simulink model "Poject_PilotInLoop_Beech_99_Nonlinear_Simulation_Altitude_hold"  (R2018b)
settings: Solver=FixedStepAuto  StartTime=0.0  StopTime=2144  FixedStep=0.01  RelTol=1e-3
InitFcn:
  | Initial_Data_Altitude_Hold
StopFcn:
  | Plots_Altitude_Hold
values from neighbouring files (symbols this model uses):
  b = 46    [Initial_Data_Altitude_Hold.m]    (also in TrimFunc.m)
  c = 6.5    [Initial_Data_Altitude_Hold.m]    (also in TrimFunc.m)
  CD0 = 0.0270    (= 0.027)    [Initial_Data_Altitude_Hold.m]    (also in TrimFunc.m)
  CDalpha = 0.131    [Initial_Data_Altitude_Hold.m]    (also in TrimFunc.m)
  CDalphadot = 0    [Initial_Data_Altitude_Hold.m]
  CDdelE = 0    [Initial_Data_Altitude_Hold.m]    (also in TrimFunc.m)
  CDiH = 0    [Initial_Data_Altitude_Hold.m]    (also in TrimFunc.m)
  CDq = 0    [Initial_Data_Altitude_Hold.m]
  CDu = 0    [Initial_Data_Altitude_Hold.m]
  CL0 = 0.201    [Initial_Data_Altitude_Hold.m]    (also in TrimFunc.m)
  CLalpha = 5.48    [Initial_Data_Altitude_Hold.m]    (also in TrimFunc.m)
  CLalphadot = 2.5    [Initial_Data_Altitude_Hold.m]
  Clbeta = -0.13    [Initial_Data_Altitude_Hold.m]    (also in TrimFunc.m)
  Clbetadot = 0    [Initial_Data_Altitude_Hold.m]
  CldelA = 0.156    [Initial_Data_Altitude_Hold.m]
  CLdelE = 0.60    (= 0.6)    [Initial_Data_Altitude_Hold.m]    (also in TrimFunc.m)
  CldelR = 0.0106    [Initial_Data_Altitude_Hold.m]    (also in TrimFunc.m)
  CLiH = 1.35    [Initial_Data_Altitude_Hold.m]    (also in TrimFunc.m)
  Clp = -0.50    (= -0.5)    [Initial_Data_Altitude_Hold.m]
  CLq = 8.1    [Initial_Data_Altitude_Hold.m]
  Clr = 0.14    [Initial_Data_Altitude_Hold.m]
  ClT = 0    [Initial_Data_Altitude_Hold.m]
  CLu = 0.020    (= 0.02)    [Initial_Data_Altitude_Hold.m]
  Cm0 = 0.05    [Initial_Data_Altitude_Hold.m]    (also in TrimFunc.m)
  Cmalpha = -1.89    [Initial_Data_Altitude_Hold.m]    (also in TrimFunc.m)
  Cmalphadot = -9.1    [Initial_Data_Altitude_Hold.m]
  CmdelE = -2.0    (= -2)    [Initial_Data_Altitude_Hold.m]    (also in TrimFunc.m)
  cmiH = -4.1    [Initial_Data_Altitude_Hold.m]
  Cmq = -34.0    (= -34)    [Initial_Data_Altitude_Hold.m]
  CmT1 = 0    [Initial_Data_Altitude_Hold.m]
  CmTalpha = 0    [Initial_Data_Altitude_Hold.m]
  CmTu = 0    [Initial_Data_Altitude_Hold.m]
  Cmu = 0    [Initial_Data_Altitude_Hold.m]
  Cnbeta = 0.080    (= 0.08)    [Initial_Data_Altitude_Hold.m]    (also in TrimFunc.m)
  Cnbetadot = 0    [Initial_Data_Altitude_Hold.m]
  CndelA = -0.0012    [Initial_Data_Altitude_Hold.m]    (also in TrimFunc.m)
  CndelR = -0.0758    [Initial_Data_Altitude_Hold.m]    (also in TrimFunc.m)
  Cnp = 0.019    [Initial_Data_Altitude_Hold.m]
  Cnr = -0.197    [Initial_Data_Altitude_Hold.m]
  CnTbeta = 0    [Initial_Data_Altitude_Hold.m]
  CTxu = -0.0596    [Initial_Data_Altitude_Hold.m]
  CTy = 0    [Initial_Data_Altitude_Hold.m]
  CTz = 0    [Initial_Data_Altitude_Hold.m]
  Cybeta = -0.59    [Initial_Data_Altitude_Hold.m]
  Cybetadot = 0    [Initial_Data_Altitude_Hold.m]
  CydelA = 0    [Initial_Data_Altitude_Hold.m]
  CydelR = 0.144    [Initial_Data_Altitude_Hold.m]
  Cyp = -0.19    [Initial_Data_Altitude_Hold.m]
  Cyr = 0.39    [Initial_Data_Altitude_Hold.m]
  delE = 0.0077075    [Initial_Data_Altitude_Hold.m]
  g = 32.17    [Initial_Data_Altitude_Hold.m]
  iH = 0    [Initial_Data_Altitude_Hold.m]    (also in TrimFunc.m)
  Ixx = 15189    [Initial_Data_Altitude_Hold.m]
  Ixz = 4371    [Initial_Data_Altitude_Hold.m]
  Iyy = 20250    [Initial_Data_Altitude_Hold.m]
  Izz = 34141    [Initial_Data_Altitude_Hold.m]
  Kp = 1    [Initial_Data_Altitude_Hold.m]
  mass = 341.9    [Initial_Data_Altitude_Hold.m]
  Ro = 0.0013    [Initial_Data_Altitude_Hold.m]
  S = 280    [Initial_Data_Altitude_Hold.m]    (also in TrimFunc.m)
  T1 = 1055.4173    [Initial_Data_Altitude_Hold.m]
  taw = 0.1    [Initial_Data_Altitude_Hold.m]
  TI = 0.2    [Initial_Data_Altitude_Hold.m]
  TL = 0.4    [Initial_Data_Altitude_Hold.m]
  TN = 0.1    [Initial_Data_Altitude_Hold.m]
libraries: simulink x1
(part 1 of 2)
settings Model: Creator=Mehdi RJ  LastModifiedBy=User
settings DataIOCC: LimitDataPoints=on  SaveFormat=Array  SignalLoggingSaveFormat=ModelDataLogs
settings OptimizationCC: BlockReduction=off  BooleanDataType=off  LifeSpan=inf
settings DebuggingCC: SaveWithParameterizedLinksMsg=none  UnderspecifiedInitializationDetection=Classic  MergeDetectMultiDrivingBlocksExec=none  SignalResolutionControl=TryResolveAllWithWarning  MultiTaskDSMMsg=warning  MultiTaskCondExecSysMsg=none  SFUnexpectedBacktrackingDiag=warning  SFNoUnconditionalDefaultTransitionDiag=warning  SFExecutionAtInitializationDiag=none
settings HardwareCC: ProdBitPerPointer=32  ProdBitPerSizeT=32  ProdBitPerPtrDiffT=32  ProdLargestAtomicFloat=None  ProdIntDivRoundTo=Undefined  ProdEndianess=Unspecified  ProdWordSize=32  ProdHWDeviceType=32-bit Generic  TargetUnknown=on
settings ModelReferenceCC: PropagateSignalLabelsOutOfModel=off
settings SFSimCC: SimUseLocalCustomCode=off
settings RTWCC: RTWUseLocalCustomCode=off
settings CodeAppCC: StateflowObjectComments=on
settings GRTTargetCC: TargetLangStandard=C89/C90 (ANSI)  GeneratePreprocessorConditionals=Disable all
settings ConfigComp: CovMetricSettings=dw  CovHtmlReporting=on  CovSaveCumulativeToWorkspaceVar=on  CovSaveSingleToWorkspaceVar=on  CovExternalEMLEnable=off

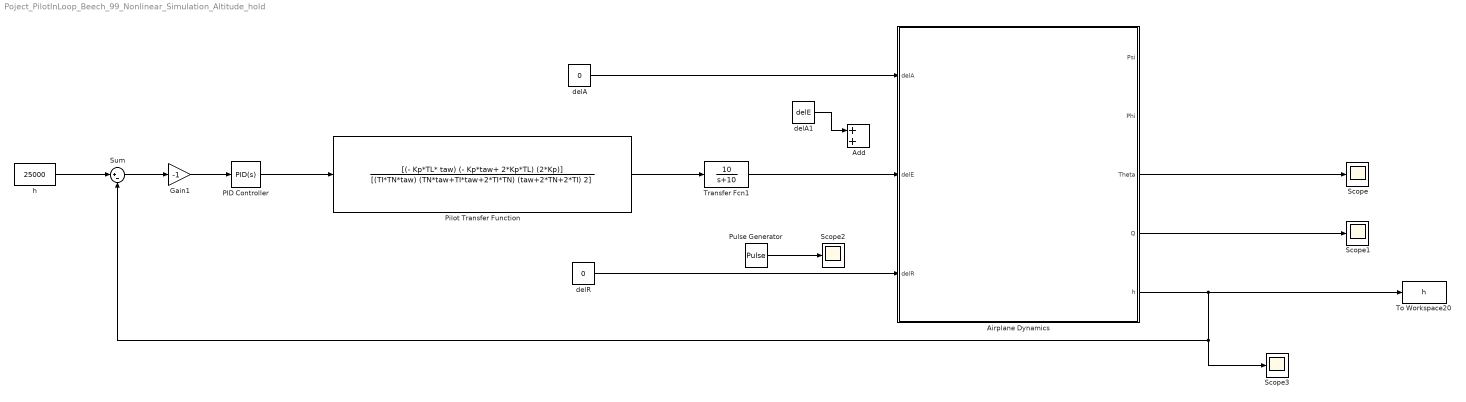
== system Poject_PilotInLoop_Beech_99_Nonlinear_Simulation_Altitude_hold ==
  Add : Sum
  Airplane Dynamics : Subsystem
  Gain1 : Gain  Gain=-1
  PID Controller : simulink/Continuous/PID Controller  Controller=PID  Form=Parallel  TimeDomain=Continuous-time  SampleTime=-1  IntegratorMethod=Forward Euler  FilterMethod=Forward Euler  ControllerParametersSource=internal  P=9.72091586765638e-06  I=5.86209894111036e-08  D=9.64251086658951e-05  UseFilter=on  N=15.2377063472214  TunerSelectOption=Transfer Function Based (PID Tuner App)  InitialConditionSource=internal  InitialConditionForIntegrator=0  InitialConditionForFilter=0  DifferentiatorICPrevScaledInput=0  ExternalReset=none  TrackingMode=off  Kt=1  LimitOutput=off  UpperSaturationLimit=inf  LowerSaturationLimit=-inf  LinearizeAsGain=on  AntiWindupMode=none  Kb=1  POutMin=[]  POutMax=[]  IOutMin=[]  IOutMax=[]  DOutMin=[]  DOutMax=[]  NOutMin=[]  NOutMax=[]  SumOutMin=[]  SumOutMax=[]  SaturationOutMin=[]  SaturationOutMax=[]  PParamMin=[]  PParamMax=[]  IParamMin=[]  IParamMax=[]  DParamMin=[]  DParamMax=[]  NParamMin=[]  NParamMax=[]  KbParamMin=[]  KbParamMax=[]  KtParamMin=[]  KtParamMax=[]  KbOutMin=[]  KbOutMax=[]  KtOutMin=[]  KtOutMax=[]  IntegratorOutMin=[]  IntegratorOutMax=[]  FilterOutMin=[]  FilterOutMax=[]  SumI1OutMin=[]  SumI1OutMax=[]  SumI2OutMin=[]  SumI2OutMax=[]  SumI3OutMin=[]  SumI3OutMax=[]  SumI4OutMin=[]  SumI4OutMax=[]  SumDOutMin=[]  SumDOutMax=[]  DifferentiatorOutMin=[]  DifferentiatorOutMax=[]  FilterDiffOutCoefMin=[]  FilterDiffOutCoefMax=[]  ReciprocalOutMin=[]  ReciprocalOutMax=[]  SumDenOutMin=[]  SumDenOutMax=[]  SumNumOutMin=[]  SumNumOutMax=[]  DivideOutMin=[]  DivideOutMax=[]  IntegratorContinuousStateAttributes=''  IntegratorStateMustResolveToSignalObject=off  IntegratorRTWStateStorageClass=Auto  FilterContinuousStateAttributes=''  FilterStateMustResolveToSignalObject=off  FilterRTWStateStorageClass=Auto  ParallelPVariant=InternalParameters  IdealPVariant=Disabled  IVariant=InternalParameters  DVariant=InternalParameters  IntegratorVariant=Continuous  SatVariant=Disabled  AWVariant=Passthrough  PCopyVariant=Disabled  TRVariant=Disabled  FdbkBlocksVariant=Forward  IdealPFdbkVariant=Disabled  SatFdbkVariant=Disabled  DerivativeFilterVariant=ContFilter  NVariant=InternalParameters  NCopyVariant=Disabled  FilterICVariant=InternalICsFilter  IntegratorICVariant=InternalICs  ExternalResetVariant=Disabled  TRSumVariant=Passthrough  SumFdbkVariant=Disabled  SumVariant=Sum_PID
  Pilot Transfer Function : TransferFcn  Numerator=[(- Kp*TL* taw) (- Kp*taw+ 2*Kp*TL) (2*Kp)]  Denominator=[(TI*TN*taw) (TN*taw+TI*taw+2*TI*TN) (taw+2*TN+2*TI) 2]
  Pulse Generator : DiscretePulseGenerator  PulseType=Time based  Amplitude=0.0175*5  Period=2000  PhaseDelay=800
  Scope{,1..3} (4 alike) : Scope
  Sum : Sum  Inputs=|+-
  To Workspace20 : ToWorkspace  VariableName=h  SampleTime=-1
  Transfer Fcn1 : TransferFcn  Numerator=[10]  Denominator=[1 10]
  delA : Constant  Value=0
  delA1 : Constant  Value=delE
  delR : Constant  Value=0
  h : Constant  Value=25000
  wires:
  delR/1 -> Airplane Dynamics/3(delR)
  delA/1 -> Airplane Dynamics/1(delA)
  Airplane Dynamics/3(Theta) -> Scope/1
  h/1 -> Sum/1
  Airplane Dynamics/4(Q) -> Scope1/1
  Pulse Generator/1 -> Scope2/1
  Sum/1 -> Gain1/1
  Gain1/1 -> PID Controller/1
  Airplane Dynamics/5(h) -> Sum/2, Scope3/1, To Workspace20/1
  Pilot Transfer Function/1 -> Transfer Fcn1/1
  PID Controller/1 -> Pilot Transfer Function/1
  delA1/1 -> Add/1
  Transfer Fcn1/1 -> Airplane Dynamics/2(delE)

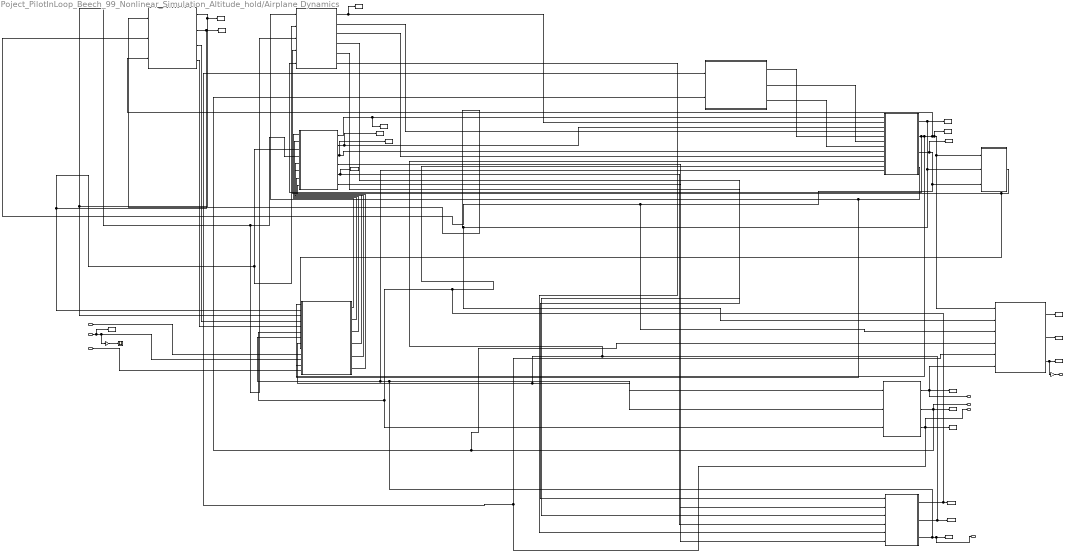
== system Poject_PilotInLoop_Beech_99_Nonlinear_Simulation_Altitude_hold/Airplane Dynamics ==
  delA : Inport
  delE : Inport  Port=2
  delR : Inport  Port=3
  AnglesBlock : Subsystem
  Angular Velocities (P,Q,R) : Subsystem
  Body Aerodynamic Forces and Moments (FAxB,FAyB,FAzB,LAB,MAB,NAB) : Subsystem
  Dynamic Pressure : Subsystem
  Euler's Angles (Phi,Theta,Psi) : Subsystem
  GBlock : Subsystem
  Gain : Gain  Gain=-1
  Gain1 : Gain  Gain=180/pi
  Linear Velocities (U,V,W) : Subsystem
  Navigation : Subsystem
  Scope : Scope
  Stability Aerodunamic Forces and Moments (FAxS,FAyS,FAzS,LAS,MAS,NAS) : Subsystem
  Thrust Forces and Moments (FTx,FTy,FTz,LT,MT,NT) : Subsystem
  To Workspace : ToWorkspace  VariableName=XInertia  SampleTime=-1
  To Workspace1 : ToWorkspace  VariableName=YInertia  SampleTime=-1
  To Workspace10 : ToWorkspace  VariableName=Q  SaveFormat=Timeseries  SampleTime=-1
  To Workspace11 : ToWorkspace  VariableName=R  SaveFormat=Timeseries  SampleTime=-1
  To Workspace12 : ToWorkspace  VariableName=P  SaveFormat=Timeseries  SampleTime=-1
  To Workspace13 : ToWorkspace  VariableName=W  SaveFormat=Timeseries  SampleTime=-1
  To Workspace14 : ToWorkspace  VariableName=FAzB  SaveFormat=Timeseries  SampleTime=-1
  To Workspace15 : ToWorkspace  VariableName=FTx  SaveFormat=Timeseries  SampleTime=-1
  To Workspace16 : ToWorkspace  VariableName=FAxB  SaveFormat=Timeseries  SampleTime=-1
  To Workspace17 : ToWorkspace  VariableName=FAyB  SaveFormat=Timeseries  SampleTime=-1
  To Workspace18 : ToWorkspace  VariableName=V  SaveFormat=Timeseries  SampleTime=-1
  To Workspace19 : ToWorkspace  VariableName=delE  SaveFormat=Timeseries  SampleTime=-1
  To Workspace2 : ToWorkspace  VariableName=ZInertia  SaveFormat=Timeseries  SampleTime=-1
  To Workspace3 : ToWorkspace  VariableName=alpha  SaveFormat=Timeseries  SampleTime=-1
  To Workspace4 : ToWorkspace  VariableName=beta  SaveFormat=Timeseries  SampleTime=-1
  To Workspace5 : ToWorkspace  VariableName=U  SaveFormat=Timeseries  SampleTime=-1
  To Workspace6 : ToWorkspace  VariableName=Psi  SaveFormat=Timeseries  SampleTime=-1
  To Workspace7 : ToWorkspace  VariableName=Phi  SaveFormat=Timeseries  SampleTime=-1
  To Workspace8 : ToWorkspace  VariableName=Theta  SaveFormat=Timeseries  SampleTime=-1
  To Workspace9 : ToWorkspace  VariableName=MAB  SaveFormat=Timeseries  SampleTime=-1
  Psi : Outport
  Phi : Outport  Port=2
  Theta : Outport  Port=3
  Q : Outport  Port=4
  h : Outport  Port=5
  wires:
  AnglesBlock/2(alpha) -> To Workspace3/1, Thrust Forces and Moments (FTx,FTy,FTz,LT,MT,NT)/2(alpha), Body Aerodynamic Forces and Moments (FAxB,FAyB,FAzB,LAB,MAB,NAB)/3(alpha), Stability Aerodunamic Forces and Moments (FAxS,FAyS,FAzS,LAS,MAS,NAS)/2(alpha)
  Stability Aerodunamic Forces and Moments (FAxS,FAyS,FAzS,LAS,MAS,NAS)/1(FAxS) -> Body Aerodynamic Forces and Moments (FAxB,FAyB,FAzB,LAB,MAB,NAB)/1(FAxS)
  Thrust Forces and Moments (FTx,FTy,FTz,LT,MT,NT)/2(FTy) -> Linear Velocities (U,V,W)/4(FTy)
  Thrust Forces and Moments (FTx,FTy,FTz,LT,MT,NT)/5(MT) -> Angular Velocities (P,Q,R)/3(MT)
  Angular Velocities (P,Q,R)/1(P) -> To Workspace12/1, Linear Velocities (U,V,W)/11(P), Stability Aerodunamic Forces and Moments (FAxS,FAyS,FAzS,LAS,MAS,NAS)/6(P), Euler's Angles (Phi,Theta,Psi)/3(P)
  AnglesBlock/3(betadot) -> Stability Aerodunamic Forces and Moments (FAxS,FAyS,FAzS,LAS,MAS,NAS)/4("betadot ")
  Euler's Angles (Phi,Theta,Psi)/1(Psi) -> To Workspace6/1, Navigation/6(Psi), Psi/1
  delR/1 -> Stability Aerodunamic Forces and Moments (FAxS,FAyS,FAzS,LAS,MAS,NAS)/13(delR)
  Body Aerodynamic Forces and Moments (FAxB,FAyB,FAzB,LAB,MAB,NAB)/4(LAB) -> Angular Velocities (P,Q,R)/2(LAB)
  Body Aerodynamic Forces and Moments (FAxB,FAyB,FAzB,LAB,MAB,NAB)/5(MAB) -> To Workspace9/1, Angular Velocities (P,Q,R)/4(MAB)
  Linear Velocities (U,V,W)/3(W) -> To Workspace13/1, Dynamic Pressure/3(W), AnglesBlock/2(W), Navigation/3(W)
  Angular Velocities (P,Q,R)/3(Q) -> Euler's Angles (Phi,Theta,Psi)/2(Q), Linear Velocities (U,V,W)/12(Q), Stability Aerodunamic Forces and Moments (FAxS,FAyS,FAzS,LAS,MAS,NAS)/7(Q), Q/1, To Workspace10/1
  Linear Velocities (U,V,W)/1(V) -> To Workspace18/1, Dynamic Pressure/2(V), AnglesBlock/1(V), Navigation/2(V)
  Euler's Angles (Phi,Theta,Psi)/3(Theta) -> To Workspace8/1, GBlock/1(Theta), Navigation/5(Theta), Theta/1
  AnglesBlock/1("beta ") -> To Workspace4/1, Body Aerodynamic Forces and Moments (FAxB,FAyB,FAzB,LAB,MAB,NAB)/4(beta), Thrust Forces and Moments (FTx,FTy,FTz,LT,MT,NT)/3(beta), Stability Aerodunamic Forces and Moments (FAxS,FAyS,FAzS,LAS,MAS,NAS)/3(beta)
  Linear Velocities (U,V,W)/4(delU) -> Stability Aerodunamic Forces and Moments (FAxS,FAyS,FAzS,LAS,MAS,NAS)/1(delU), Thrust Forces and Moments (FTx,FTy,FTz,LT,MT,NT)/1(delU)
  Thrust Forces and Moments (FTx,FTy,FTz,LT,MT,NT)/3(FTz) -> Linear Velocities (U,V,W)/9(FTz)
  Navigation/2(YInertia) -> To Workspace1/1
  Stability Aerodunamic Forces and Moments (FAxS,FAyS,FAzS,LAS,MAS,NAS)/4(LAS) -> Body Aerodynamic Forces and Moments (FAxB,FAyB,FAzB,LAB,MAB,NAB)/6(LAS)
  Euler's Angles (Phi,Theta,Psi)/2(Phi) -> To Workspace7/1, Navigation/4(Phi), GBlock/2("Phi "), Phi/1
  Body Aerodynamic Forces and Moments (FAxB,FAyB,FAzB,LAB,MAB,NAB)/3(FAzB) -> To Workspace14/1, Linear Velocities (U,V,W)/8(FAzB)
  Stability Aerodunamic Forces and Moments (FAxS,FAyS,FAzS,LAS,MAS,NAS)/2(FAyS) -> Body Aerodynamic Forces and Moments (FAxB,FAyB,FAzB,LAB,MAB,NAB)/2(FAyS)
  GBlock/2(gy) -> Linear Velocities (U,V,W)/6(gy)
  AnglesBlock/4(alphadot) -> Stability Aerodunamic Forces and Moments (FAxS,FAyS,FAzS,LAS,MAS,NAS)/5(alphadot)
  Navigation/1(XInertia) -> To Workspace/1
  Thrust Forces and Moments (FTx,FTy,FTz,LT,MT,NT)/1(FTx) -> To Workspace15/1, Linear Velocities (U,V,W)/2(FTx)
  Stability Aerodunamic Forces and Moments (FAxS,FAyS,FAzS,LAS,MAS,NAS)/5(MAS) -> Body Aerodynamic Forces and Moments (FAxB,FAyB,FAzB,LAB,MAB,NAB)/7(MAS)
  Thrust Forces and Moments (FTx,FTy,FTz,LT,MT,NT)/6(NT) -> Angular Velocities (P,Q,R)/5(NT)
  Stability Aerodunamic Forces and Moments (FAxS,FAyS,FAzS,LAS,MAS,NAS)/6(NAS) -> Body Aerodynamic Forces and Moments (FAxB,FAyB,FAzB,LAB,MAB,NAB)/8(NAS)
  Navigation/3(ZInertia) -> Gain/1, To Workspace2/1
  Linear Velocities (U,V,W)/2(U) -> Thrust Forces and Moments (FTx,FTy,FTz,LT,MT,NT)/5(U), Stability Aerodunamic Forces and Moments (FAxS,FAyS,FAzS,LAS,MAS,NAS)/12(U), AnglesBlock/3(U), To Workspace5/1, Navigation/1(U), Dynamic Pressure/1(U)
  Stability Aerodunamic Forces and Moments (FAxS,FAyS,FAzS,LAS,MAS,NAS)/3(FAzS) -> Body Aerodynamic Forces and Moments (FAxB,FAyB,FAzB,LAB,MAB,NAB)/5(FAzS)
  Dynamic Pressure/1(q1) -> Stability Aerodunamic Forces and Moments (FAxS,FAyS,FAzS,LAS,MAS,NAS)/9(q1), Thrust Forces and Moments (FTx,FTy,FTz,LT,MT,NT)/4(q1)
  Body Aerodynamic Forces and Moments (FAxB,FAyB,FAzB,LAB,MAB,NAB)/6(NAB) -> Angular Velocities (P,Q,R)/6(NAB)
  GBlock/1(gx) -> Linear Velocities (U,V,W)/5(gx)
  GBlock/3(gz) -> Linear Velocities (U,V,W)/7(gz)
  Body Aerodynamic Forces and Moments (FAxB,FAyB,FAzB,LAB,MAB,NAB)/1(FAxB) -> To Workspace16/1, Linear Velocities (U,V,W)/1(FAxB)
  Angular Velocities (P,Q,R)/2(R) -> To Workspace11/1, Stability Aerodunamic Forces and Moments (FAxS,FAyS,FAzS,LAS,MAS,NAS)/8(R), Euler's Angles (Phi,Theta,Psi)/1(R), Linear Velocities (U,V,W)/10(R)
  Thrust Forces and Moments (FTx,FTy,FTz,LT,MT,NT)/4(LT) -> Angular Velocities (P,Q,R)/1(LT)
  Body Aerodynamic Forces and Moments (FAxB,FAyB,FAzB,LAB,MAB,NAB)/2(FAyB) -> To Workspace17/1, Linear Velocities (U,V,W)/3(FAyB)
  delA/1 -> Stability Aerodunamic Forces and Moments (FAxS,FAyS,FAzS,LAS,MAS,NAS)/10(delA)
  Gain/1 -> h/1
  delE/1 -> To Workspace19/1, Gain1/1, Stability Aerodunamic Forces and Moments (FAxS,FAyS,FAzS,LAS,MAS,NAS)/11(delE)
  Gain1/1 -> Scope/1

== system Poject_PilotInLoop_Beech_99_Nonlinear_Simulation_Altitude_hold/Airplane Dynamics/AnglesBlock ==
  V : Inport
  W : Inport  Port=2
  U : Inport  Port=3
  Atan2 : Trigonometry  Operator=atan2
  Derivative : Derivative
  Derivative1 : Derivative
  Divide : Product  Inputs=*/
  Scope : Scope
  Sin : Trigonometry  Operator=asin
  "beta " : Outport
  alpha : Outport  Port=2
  betadot : Outport  Port=3
  alphadot : Outport  Port=4
  wires:
  U/1 -> Atan2/2, Divide/2
  W/1 -> Atan2/1
  V/1 -> Divide/1
  Atan2/1 -> Derivative1/1, Scope/1, alpha/1
  Sin/1 -> Derivative/1, "beta "/1
  Divide/1 -> Sin/1
  Derivative/1 -> betadot/1
  Derivative1/1 -> alphadot/1

== system Poject_PilotInLoop_Beech_99_Nonlinear_Simulation_Altitude_hold/Airplane Dynamics/Angular Velocities (P,Q,R) ==
  LT : Inport
  LAB : Inport  Port=2
  MT : Inport  Port=3
  MAB : Inport  Port=4
  NT : Inport  Port=5
  NAB : Inport  Port=6
  PBlock : Subsystem
  QBlock : Subsystem
  RBlock : Subsystem
  Scope : Scope
  P : Outport
  R : Outport  Port=2
  Q : Outport  Port=3
  wires:
  PBlock/2(Pdot) -> RBlock/3(Pdot)
  PBlock/1(P) -> RBlock/5(P), QBlock/3(P), P/1
  RBlock/2("Rdot ") -> PBlock/3(Rdot)
  LT/1 -> PBlock/2(LT)
  MAB/1 -> QBlock/1(MAB)
  LAB/1 -> PBlock/1(LAB)
  RBlock/1(R) -> R/1, PBlock/4(R), QBlock/4(R)
  NAB/1 -> RBlock/1(NAB)
  NT/1 -> RBlock/2(NT)
  MT/1 -> QBlock/2(MT)
  QBlock/1(Q) -> PBlock/5(Q), RBlock/4(Q), Scope/1, Q/1

== system Poject_PilotInLoop_Beech_99_Nonlinear_Simulation_Altitude_hold/Airplane Dynamics/Body Aerodynamic Forces and Moments (FAxB,FAyB,FAzB,LAB,MAB,NAB) ==
  FAxS : Inport
  FAyS : Inport  Port=2
  alpha : Inport  Port=3
  beta : Inport  Port=4
  FAzS : Inport  Port=5
  LAS : Inport  Port=6
  MAS : Inport  Port=7
  NAS : Inport  Port=8
  FAxBBlock : Subsystem
  FAyBBlock : Subsystem
  FAzBBlock : Subsystem
  LABBlock : Subsystem
  MABBlock : Subsystem
  NABBlock : Subsystem
  FAxB : Outport
  FAyB : Outport  Port=2
  FAzB : Outport  Port=3
  LAB : Outport  Port=4
  MAB : Outport  Port=5
  NAB : Outport  Port=6
  wires:
  LAS/1 -> NABBlock/1(LAS), MABBlock/1(LAS), LABBlock/1(LAS)
  NAS/1 -> NABBlock/3(NAS), LABBlock/3(NAS)
  MAS/1 -> NABBlock/2(MAS), LABBlock/2(MAS), MABBlock/2(MAS)
  FAyS/1 -> FAzBBlock/2(FAyS), FAyBBlock/2(FAyS), FAxBBlock/2(FAyS)
  beta/1 -> MABBlock/3(beta), FAxBBlock/5(beta), FAyBBlock/3(beta), FAzBBlock/5(beta), NABBlock/5(beta), LABBlock/5(beta)
  FAzS/1 -> FAxBBlock/3(FAzS), FAzBBlock/3(FAzS)
  MABBlock/1(MAB) -> MAB/1
  FAxS/1 -> FAyBBlock/1(FAxS), FAzBBlock/1(FAxS), FAxBBlock/1(FAxS)
  NABBlock/1(NAB) -> NAB/1
  LABBlock/1(LAB) -> LAB/1
  alpha/1 -> FAzBBlock/4(alpha), FAxBBlock/4(alpha), NABBlock/4(alpha), LABBlock/4(alpha)
  FAxBBlock/1(FAxB) -> FAxB/1
  FAyBBlock/1(FAyB) -> FAyB/1
  FAzBBlock/1(FAzB) -> FAzB/1

== system Poject_PilotInLoop_Beech_99_Nonlinear_Simulation_Altitude_hold/Airplane Dynamics/Dynamic Pressure ==
  U : Inport
  V : Inport  Port=2
  W : Inport  Port=3
  Add : Sum  Inputs=+++
  Constant : Constant  Value=2
  Constant1 : Constant  Value=2
  Constant2 : Constant  Value=2
  Divide : Product  Inputs=**/
  Divide1 : Product  Inputs=**/
  Divide2 : Product  Inputs=**/
  Multiply : Product
  Multiply1 : Product
  Multiply2 : Product
  Ro : Constant  Value=Ro
  Ro1 : Constant  Value=Ro
  Ro2 : Constant  Value=Ro
  q1 : Outport
  wires:
  Constant2/1 -> Divide2/3
  Add/1 -> q1/1
  Multiply2/1 -> Divide2/2
  V/1 -> Multiply1/1, Multiply1/2
  Divide2/1 -> Add/3
  Constant/1 -> Divide/3
  Multiply1/1 -> Divide1/2
  Divide1/1 -> Add/2
  U/1 -> Multiply/2, Multiply/1
  Ro2/1 -> Divide2/1
  Multiply/1 -> Divide/2
  W/1 -> Multiply2/1, Multiply2/2
  Divide/1 -> Add/1
  Ro1/1 -> Divide1/1
  Constant1/1 -> Divide1/3
  Ro/1 -> Divide/1

== system Poject_PilotInLoop_Beech_99_Nonlinear_Simulation_Altitude_hold/Airplane Dynamics/Euler's Angles (Phi,Theta,Psi) ==
  R : Inport
  Q : Inport  Port=2
  P : Inport  Port=3
  PhiBlock : Subsystem
  PsiBlock : Subsystem
  ThetaBlock : Subsystem
  Psi : Outport
  Phi : Outport  Port=2
  Theta : Outport  Port=3
  wires:
  P/1 -> PhiBlock/1(P)
  ThetaBlock/1(Theta) -> PhiBlock/3(Theta), Theta/1, PsiBlock/3("Theta ")
  PhiBlock/1(Phi) -> PsiBlock/2("Phi "), ThetaBlock/1(Phi), Phi/1
  Q/1 -> PsiBlock/1(Q), ThetaBlock/3(Q), PhiBlock/2(Q)
  R/1 -> PsiBlock/4("R "), ThetaBlock/2(R), PhiBlock/4(R)
  PsiBlock/1(Psi) -> Psi/1

== system Poject_PilotInLoop_Beech_99_Nonlinear_Simulation_Altitude_hold/Airplane Dynamics/GBlock ==
  Theta : Inport
  "Phi " : Inport  Port=2
  Cos : Trigonometry  Operator=cos
  Cos1 : Trigonometry  Operator=cos
  Gain : Gain  Gain=-1
  "Gravityl Acceleration " : Constant  Value=g
  Multiply : Product
  Multiply1 : Product  Inputs=3
  Multiply2 : Product  Inputs=3
  Scope : Scope
  Scope1 : Scope
  Scope2 : Scope
  Trigonometric Function : Trigonometry
  Trigonometric Function1 : Trigonometry
  gx : Outport
  gy : Outport  Port=2
  gz : Outport  Port=3
  wires:
  Multiply2/1 -> Scope2/1, gz/1
  "Gravityl Acceleration "/1 -> Multiply1/1, Multiply2/1, Multiply/2
  Theta/1 -> Cos1/1, Trigonometric Function/1
  "Phi "/1 -> Trigonometric Function1/1, Cos/1
  Multiply/1 -> Scope/1, gx/1
  Multiply1/1 -> Scope1/1, gy/1
  Trigonometric Function1/1 -> Multiply1/2
  Cos1/1 -> Multiply2/2, Multiply1/3
  Cos/1 -> Multiply2/3
  Trigonometric Function/1 -> Gain/1
  Gain/1 -> Multiply/1

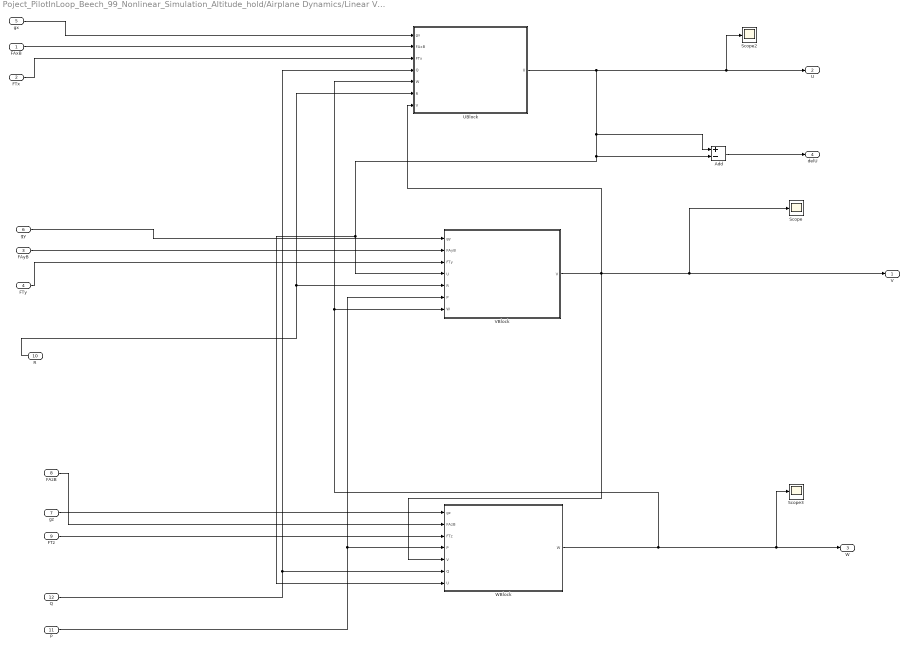
== system Poject_PilotInLoop_Beech_99_Nonlinear_Simulation_Altitude_hold/Airplane Dynamics/Linear Velocities (U,V,W) ==
  FAxB : Inport
  FTx : Inport  Port=2
  FAyB : Inport  Port=3
  FTy : Inport  Port=4
  gx : Inport  Port=5
  gy : Inport  Port=6
  gz : Inport  Port=7
  FAzB : Inport  Port=8
  FTz : Inport  Port=9
  R : Inport  Port=10
  P : Inport  Port=11
  Q : Inport  Port=12
  Add : Sum  Inputs=+-
  Scope : Scope
  Scope2 : Scope
  Scope3 : Scope
  UBlock : Subsystem
  VBlock : Subsystem
  WBlock : Subsystem
  V : Outport
  U : Outport  Port=2
  W : Outport  Port=3
  delU : Outport  Port=4
  wires:
  VBlock/1(V) -> Scope/1, V/1, WBlock/5(V), UBlock/7(V)
  FTx/1 -> UBlock/3("FTx ")
  FAxB/1 -> UBlock/2("FAxB ")
  Q/1 -> UBlock/4("Q "), WBlock/6("Q ")
  R/1 -> UBlock/6("R "), VBlock/5(R)
  FTz/1 -> WBlock/3("FTz ")
  P/1 -> VBlock/6("P "), WBlock/4("P ")
  gy/1 -> VBlock/1(gy)
  FAyB/1 -> VBlock/2("FAyB ")
  gx/1 -> UBlock/1(gx)
  FTy/1 -> VBlock/3("FTy ")
  FAzB/1 -> WBlock/2("FAzB ")
  WBlock/1(W) -> VBlock/7(W), UBlock/5(W), Scope3/1, W/1
  gz/1 -> WBlock/1(gz)
  UBlock/1(U) -> WBlock/7("U "), VBlock/4("U "), Add/2, Add/1, Scope2/1, U/1
  Add/1 -> delU/1

== system Poject_PilotInLoop_Beech_99_Nonlinear_Simulation_Altitude_hold/Airplane Dynamics/Navigation ==
  U : Inport
  V : Inport  Port=2
  W : Inport  Port=3
  Phi : Inport  Port=4
  Theta : Inport  Port=5
  Psi : Inport  Port=6
  XInertiaBlock : Subsystem
  YInertiaBlock : Subsystem
  ZInertiaBlock : Subsystem
  XInertia : Outport
  YInertia : Outport  Port=2
  ZInertia : Outport  Port=3
  wires:
  XInertiaBlock/1(XInertia) -> XInertia/1
  Phi/1 -> ZInertiaBlock/4(Phi), YInertiaBlock/4(Phi), XInertiaBlock/4(Phi)
  ZInertiaBlock/1(ZInertia) -> ZInertia/1
  V/1 -> XInertiaBlock/2(V), YInertiaBlock/2(V), ZInertiaBlock/2(V)
  Theta/1 -> ZInertiaBlock/5(Theta), YInertiaBlock/5(Theta), XInertiaBlock/5(Theta)
  U/1 -> ZInertiaBlock/1(U), YInertiaBlock/1(U), XInertiaBlock/1(U)
  Psi/1 -> XInertiaBlock/6(Psi), YInertiaBlock/6(Psi)
  W/1 -> YInertiaBlock/3(W), ZInertiaBlock/3(W), XInertiaBlock/3(W)
  YInertiaBlock/1(YInertia) -> YInertia/1

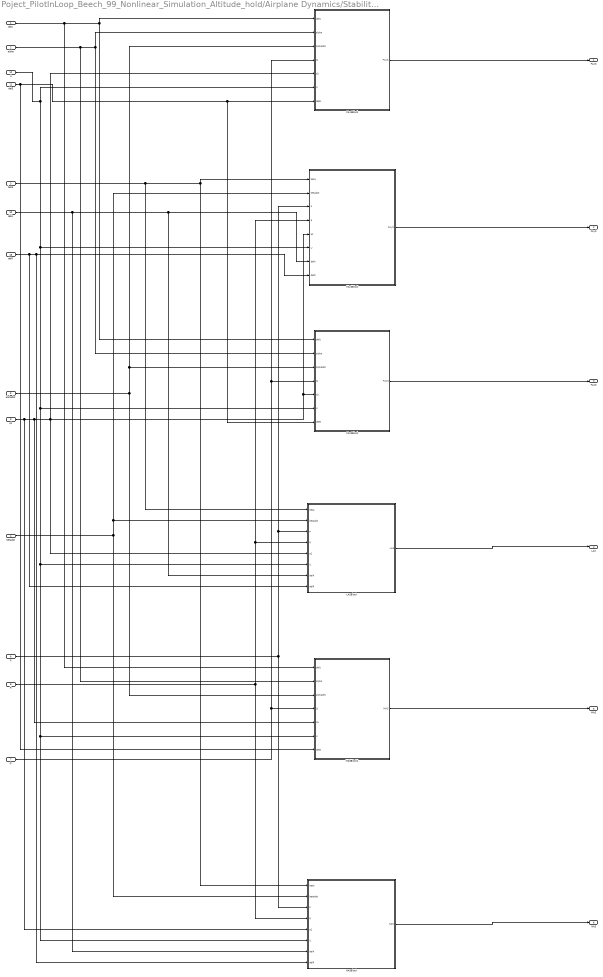
== system Poject_PilotInLoop_Beech_99_Nonlinear_Simulation_Altitude_hold/Airplane Dynamics/Stability Aerodunamic Forces and Moments (FAxS,FAyS,FAzS,LAS,MAS,NAS) ==
  delU : Inport
  alpha : Inport  Port=2
  beta : Inport  Port=3
  "betadot " : Inport  Port=4
  alphadot : Inport  Port=5
  P : Inport  Port=6
  Q : Inport  Port=7
  R : Inport  Port=8
  q1 : Inport  Port=9
  delA : Inport  Port=10
  delE : Inport  Port=11
  U : Inport  Port=12
  delR : Inport  Port=13
  FAxSBlock : Subsystem
  FAySBlock : Subsystem
  FAzSBlock : Subsystem
  LASBlock : Subsystem
  MASBlock1 : Subsystem
  NASBlock : Subsystem
  FAxS : Outport
  FAyS : Outport  Port=2
  FAzS : Outport  Port=3
  LAS : Outport  Port=4
  MAS : Outport  Port=5
  NAS : Outport  Port=6
  wires:
  LASBlock/1(LAS) -> LAS/1
  alphadot/1 -> FAxSBlock/3(alphadot), FAzSBlock/3(alphadot), MASBlock1/3(alphadot)
  P/1 -> LASBlock/3(P), FAySBlock/3(P), NASBlock/3(P)
  R/1 -> FAySBlock/4(R), LASBlock/4(R), NASBlock/4(R)
  Q/1 -> MASBlock1/4(Q), FAzSBlock/4(Q), FAxSBlock/4(Q)
  FAzSBlock/1(FAzS) -> FAzS/1
  beta/1 -> LASBlock/1(beta), NASBlock/1(beta), FAySBlock/1(beta)
  "betadot "/1 -> FAySBlock/2(betadot), LASBlock/2(betadot), NASBlock/2(betadot)
  NASBlock/1(NAS) -> NAS/1
  FAySBlock/1(FAyS) -> FAyS/1
  alpha/1 -> MASBlock1/2(alpha), FAzSBlock/2(alpha), FAxSBlock/2(alpha)
  FAxSBlock/1(FAxS) -> FAxS/1
  delU/1 -> MASBlock1/1(delU), FAzSBlock/1(delU), FAxSBlock/1(delU)
  MASBlock1/1(MAS) -> MAS/1
  q1/1 -> NASBlock/5(q1), MASBlock1/5(q1), FAzSBlock/5(q1), FAySBlock/5(q1), LASBlock/5(q1), FAxSBlock/5(q1)
  U/1 -> NASBlock/6(U), MASBlock1/6(U), LASBlock/6(U), FAzSBlock/6(U), FAySBlock/6(U), FAxSBlock/6(U)
  delE/1 -> MASBlock1/7(delE), FAzSBlock/7(delE), FAxSBlock/7(delE)
  delA/1 -> NASBlock/7(delA), LASBlock/7(delA), FAySBlock/7(delA)
  delR/1 -> LASBlock/8(delR), NASBlock/8(delR), FAySBlock/8(delR)

== system Poject_PilotInLoop_Beech_99_Nonlinear_Simulation_Altitude_hold/Airplane Dynamics/Thrust Forces and Moments (FTx,FTy,FTz,LT,MT,NT) ==
  delU : Inport
  alpha : Inport  Port=2
  beta : Inport  Port=3
  q1 : Inport  Port=4
  U : Inport  Port=5
  FTxBlock : Subsystem
  FTyBlock : Subsystem
  FTzBlock : Subsystem
  LTBlock : Subsystem
  MTBlock : Subsystem
  NTBlock : Subsystem
  FTx : Outport
  FTy : Outport  Port=2
  FTz : Outport  Port=3
  LT : Outport  Port=4
  MT : Outport  Port=5
  NT : Outport  Port=6
  wires:
  FTxBlock/1(FTx) -> FTx/1
  LTBlock/1(LT) -> LT/1
  delU/1 -> MTBlock/1(delU), FTxBlock/1(delU)
  alpha/1 -> MTBlock/2(alpha)
  FTyBlock/1(FTy) -> FTy/1
  beta/1 -> NTBlock/1(beta)
  NTBlock/1(NT) -> NT/1
  MTBlock/1(MT) -> MT/1
  FTzBlock/1(FTz) -> FTz/1
  q1/1 -> NTBlock/2(q1), MTBlock/3(q1), LTBlock/1(q1), FTzBlock/1(q1), FTyBlock/1(q1), FTxBlock/2(q1)
  U/1 -> FTxBlock/3(U), MTBlock/4(U)

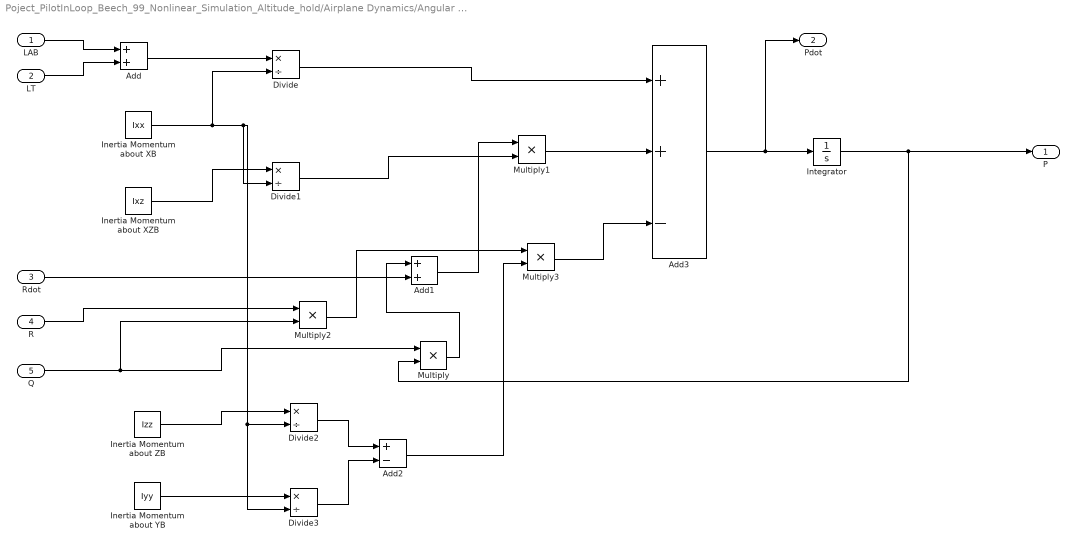
== system Poject_PilotInLoop_Beech_99_Nonlinear_Simulation_Altitude_hold/Airplane Dynamics/Angular Velocities (P,Q,R)/PBlock ==
  LAB : Inport
  LT : Inport  Port=2
  Rdot : Inport  Port=3
  R : Inport  Port=4
  Q : Inport  Port=5
  Add : Sum
  Add1 : Sum
  Add2 : Sum  Inputs=+-
  Add3 : Sum  Inputs=++-
  Divide{,1..3} (4 alike) : Product  Inputs=*/
  Inertia Momentum about XB : Constant  Value=Ixx
  Inertia Momentum about XZB : Constant  Value=Ixz
  Inertia Momentum about YB : Constant  Value=Iyy
  Inertia Momentum about ZB : Constant  Value=Izz
  Integrator : Integrator
  Multiply{,1..3} (4 alike) : Product
  P : Outport
  Pdot : Outport  Port=2
  wires:
  Integrator/1 -> Multiply/2, P/1
  LAB/1 -> Add/1
  LT/1 -> Add/2
  Add/1 -> Divide/1
  Inertia Momentum about XB/1 -> Divide1/2, Divide2/2, Divide3/2, Divide/2
  Divide/1 -> Add3/1
  Rdot/1 -> Add1/2
  Q/1 -> Multiply2/2, Multiply/1
  Multiply/1 -> Add1/1
  Inertia Momentum about XZB/1 -> Divide1/1
  Add1/1 -> Multiply1/1
  Divide1/1 -> Multiply1/2
  Multiply1/1 -> Add3/2
  R/1 -> Multiply2/1
  Inertia Momentum about ZB/1 -> Divide2/1
  Inertia Momentum about YB/1 -> Divide3/1
  Divide2/1 -> Add2/1
  Divide3/1 -> Add2/2
  Add2/1 -> Multiply3/2
  Multiply2/1 -> Multiply3/1
  Multiply3/1 -> Add3/3
  Add3/1 -> Pdot/1, Integrator/1

== system Poject_PilotInLoop_Beech_99_Nonlinear_Simulation_Altitude_hold/Airplane Dynamics/Angular Velocities (P,Q,R)/QBlock ==
  MAB : Inport
  MT : Inport  Port=2
  P : Inport  Port=3
  R : Inport  Port=4
  Add : Sum
  Add1 : Sum  Inputs=+-
  Add2 : Sum  Inputs=+-
  Add3 : Sum  Inputs=+--
  Divide1 : Product  Inputs=*/
  Divide2 : Product  Inputs=/*
  Divide3 : Product  Inputs=/*
  Inertia Momentum about XB : Constant  Value=Ixx
  Inertia Momentum about XZB : Constant  Value=Ixz
  Inertia Momentum about YB : Constant  Value=Iyy
  Inertia Momentum about ZB : Constant  Value=Izz
  Integrator : Integrator
  Multiply{,1..4} (5 alike) : Product
  Q : Outport
  wires:
  Divide2/1 -> Multiply/1
  Add3/1 -> Integrator/1
  Inertia Momentum about XZB/1 -> Divide2/2
  Divide3/1 -> Multiply2/2
  Integrator/1 -> Q/1
  Divide1/1 -> Add3/1
  Add2/1 -> Divide3/2
  MT/1 -> Add/2
  Multiply/1 -> Add3/2
  Inertia Momentum about YB/1 -> Divide3/1, Divide2/1, Divide1/2
  Add1/1 -> Multiply/2
  Multiply1/1 -> Multiply2/1
  Add/1 -> Divide1/1
  Multiply2/1 -> Add3/3
  MAB/1 -> Add/1
  Inertia Momentum about ZB/1 -> Add2/2
  Inertia Momentum about XB/1 -> Add2/1
  P/1 -> Multiply3/2, Multiply3/1, Multiply1/1
  R/1 -> Multiply4/2, Multiply1/2, Multiply4/1
  Multiply3/1 -> Add1/1
  Multiply4/1 -> Add1/2

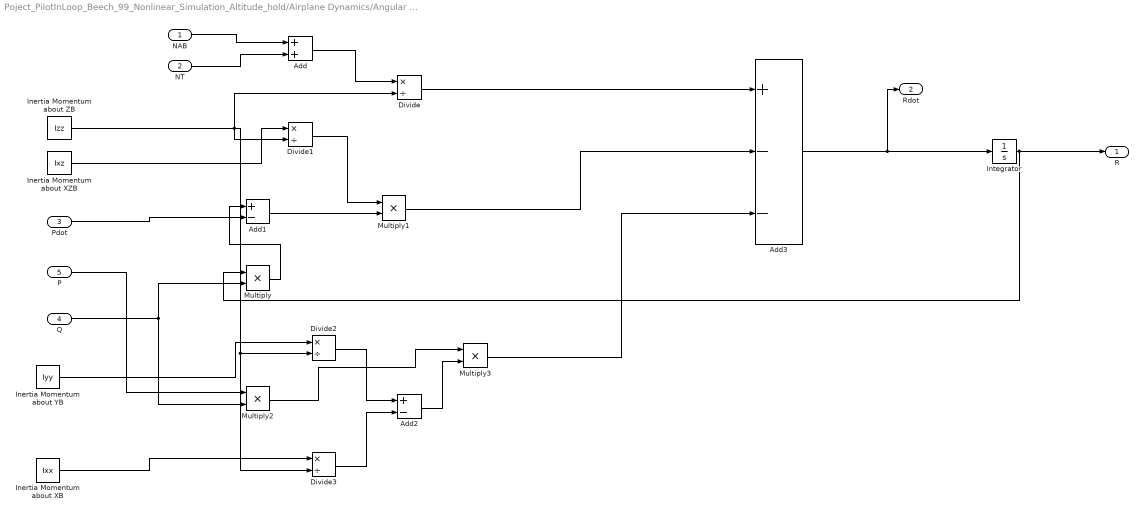
== system Poject_PilotInLoop_Beech_99_Nonlinear_Simulation_Altitude_hold/Airplane Dynamics/Angular Velocities (P,Q,R)/RBlock ==
  NAB : Inport
  NT : Inport  Port=2
  Pdot : Inport  Port=3
  Q : Inport  Port=4
  P : Inport  Port=5
  Add : Sum
  Add1 : Sum  Inputs=+-
  Add2 : Sum  Inputs=+-
  Add3 : Sum  Inputs=+--
  Divide{,1..3} (4 alike) : Product  Inputs=*/
  Inertia Momentum about XB : Constant  Value=Ixx
  Inertia Momentum about XZB : Constant  Value=Ixz
  Inertia Momentum about YB : Constant  Value=Iyy
  Inertia Momentum about ZB : Constant  Value=Izz
  Integrator : Integrator
  Multiply{,1..3} (4 alike) : Product
  R : Outport
  "Rdot " : Outport  Port=2
  wires:
  Integrator/1 -> Multiply/1, R/1
  Add3/1 -> "Rdot "/1, Integrator/1
  NAB/1 -> Add/1
  NT/1 -> Add/2
  Add/1 -> Divide/1
  Inertia Momentum about ZB/1 -> Divide2/2, Divide3/2, Divide1/2, Divide/2
  Divide/1 -> Add3/1
  Q/1 -> Multiply2/2, Multiply/2
  Multiply/1 -> Add1/1
  Pdot/1 -> Add1/2
  Add1/1 -> Multiply1/2
  Inertia Momentum about XZB/1 -> Divide1/1
  Divide1/1 -> Multiply1/1
  Multiply1/1 -> Add3/2
  P/1 -> Multiply2/1
  Inertia Momentum about YB/1 -> Divide2/1
  Inertia Momentum about XB/1 -> Divide3/1
  Divide3/1 -> Add2/2
  Divide2/1 -> Add2/1
  Multiply2/1 -> Multiply3/1
  Add2/1 -> Multiply3/2
  Multiply3/1 -> Add3/3

== system Poject_PilotInLoop_Beech_99_Nonlinear_Simulation_Altitude_hold/Airplane Dynamics/Body Aerodynamic Forces and Moments (FAxB,FAyB,FAzB,LAB,MAB,NAB)/FAxBBlock ==
  FAxS : Inport
  FAyS : Inport  Port=2
  FAzS : Inport  Port=3
  alpha : Inport  Port=4
  beta : Inport  Port=5
  Add1 : Sum  Inputs=+--
  Cos : Trigonometry  Operator=cos
  Cos1 : Trigonometry  Operator=cos
  Multiply : Product  Inputs=***
  Multiply1 : Product  Inputs=***
  Multiply2 : Product  Inputs=**
  Sin : Trigonometry
  Sin1 : Trigonometry
  FAxB : Outport
  wires:
  Add1/1 -> FAxB/1
  Multiply1/1 -> Add1/2
  FAxS/1 -> Multiply/2
  Cos1/1 -> Multiply/3
  alpha/1 -> Cos/1, Sin1/1
  FAyS/1 -> Multiply1/1
  Multiply/1 -> Add1/1
  Cos/1 -> Multiply/1, Multiply1/2
  beta/1 -> Cos1/1, Sin/1
  Sin1/1 -> Multiply2/1
  Multiply2/1 -> Add1/3
  FAzS/1 -> Multiply2/2
  Sin/1 -> Multiply1/3

== system Poject_PilotInLoop_Beech_99_Nonlinear_Simulation_Altitude_hold/Airplane Dynamics/Body Aerodynamic Forces and Moments (FAxB,FAyB,FAzB,LAB,MAB,NAB)/FAyBBlock ==
  FAxS : Inport
  FAyS : Inport  Port=2
  beta : Inport  Port=3
  Add1 : Sum
  Cos1 : Trigonometry  Operator=cos
  Multiply : Product  Inputs=**
  Multiply1 : Product  Inputs=**
  Sin : Trigonometry
  FAyB : Outport
  wires:
  Sin/1 -> Multiply1/2
  beta/1 -> Sin/1, Cos1/1
  Multiply/1 -> Add1/1
  Cos1/1 -> Multiply/2
  Multiply1/1 -> Add1/2
  Add1/1 -> FAyB/1
  FAxS/1 -> Multiply1/1
  FAyS/1 -> Multiply/1

== system Poject_PilotInLoop_Beech_99_Nonlinear_Simulation_Altitude_hold/Airplane Dynamics/Body Aerodynamic Forces and Moments (FAxB,FAyB,FAzB,LAB,MAB,NAB)/FAzBBlock ==
  FAxS : Inport
  FAyS : Inport  Port=2
  FAzS : Inport  Port=3
  alpha : Inport  Port=4
  beta : Inport  Port=5
  Add1 : Sum  Inputs=+-+
  Cos : Trigonometry  Operator=cos
  Cos1 : Trigonometry  Operator=cos
  Multiply : Product  Inputs=***
  Multiply1 : Product  Inputs=***
  Multiply2 : Product  Inputs=**
  Sin : Trigonometry
  Sin2 : Trigonometry
  FAzB : Outport
  wires:
  Add1/1 -> FAzB/1
  Multiply1/1 -> Add1/2
  FAxS/1 -> Multiply/2
  Cos1/1 -> Multiply/3
  alpha/1 -> Cos/1, Sin2/1
  FAyS/1 -> Multiply1/1
  Multiply/1 -> Add1/1
  Sin2/1 -> Multiply/1, Multiply1/2
  beta/1 -> Cos1/1, Sin/1
  Cos/1 -> Multiply2/1
  Multiply2/1 -> Add1/3
  FAzS/1 -> Multiply2/2
  Sin/1 -> Multiply1/3

== system Poject_PilotInLoop_Beech_99_Nonlinear_Simulation_Altitude_hold/Airplane Dynamics/Body Aerodynamic Forces and Moments (FAxB,FAyB,FAzB,LAB,MAB,NAB)/LABBlock ==
  LAS : Inport
  MAS : Inport  Port=2
  NAS : Inport  Port=3
  alpha : Inport  Port=4
  beta : Inport  Port=5
  Add1 : Sum  Inputs=+--
  Cos : Trigonometry  Operator=cos
  Cos1 : Trigonometry  Operator=cos
  Multiply : Product  Inputs=***
  Multiply1 : Product  Inputs=***
  Multiply2 : Product  Inputs=**
  Sin : Trigonometry
  Sin1 : Trigonometry
  LAB : Outport
  wires:
  Sin/1 -> Multiply1/3
  NAS/1 -> Multiply2/2
  Multiply2/1 -> Add1/3
  Sin1/1 -> Multiply2/1
  beta/1 -> Sin/1, Cos1/1
  Cos/1 -> Multiply1/2, Multiply/1
  Multiply/1 -> Add1/1
  MAS/1 -> Multiply1/1
  alpha/1 -> Sin1/1, Cos/1
  Cos1/1 -> Multiply/3
  LAS/1 -> Multiply/2
  Multiply1/1 -> Add1/2
  Add1/1 -> LAB/1

== system Poject_PilotInLoop_Beech_99_Nonlinear_Simulation_Altitude_hold/Airplane Dynamics/Body Aerodynamic Forces and Moments (FAxB,FAyB,FAzB,LAB,MAB,NAB)/MABBlock ==
  LAS : Inport
  MAS : Inport  Port=2
  beta : Inport  Port=3
  Add1 : Sum
  Cos1 : Trigonometry  Operator=cos
  Multiply : Product  Inputs=**
  Multiply1 : Product  Inputs=**
  Sin : Trigonometry
  MAB : Outport
  wires:
  MAS/1 -> Multiply/1
  LAS/1 -> Multiply1/1
  Add1/1 -> MAB/1
  Multiply1/1 -> Add1/2
  Cos1/1 -> Multiply/2
  Multiply/1 -> Add1/1
  beta/1 -> Cos1/1, Sin/1
  Sin/1 -> Multiply1/2

== system Poject_PilotInLoop_Beech_99_Nonlinear_Simulation_Altitude_hold/Airplane Dynamics/Body Aerodynamic Forces and Moments (FAxB,FAyB,FAzB,LAB,MAB,NAB)/NABBlock ==
  LAS : Inport
  MAS : Inport  Port=2
  NAS : Inport  Port=3
  alpha : Inport  Port=4
  beta : Inport  Port=5
  Add1 : Sum  Inputs=+-+
  Cos : Trigonometry  Operator=cos
  Cos1 : Trigonometry  Operator=cos
  Multiply : Product  Inputs=***
  Multiply1 : Product  Inputs=***
  Multiply2 : Product  Inputs=**
  Sin : Trigonometry
  Sin2 : Trigonometry
  NAB : Outport
  wires:
  Sin/1 -> Multiply1/3
  NAS/1 -> Multiply2/2
  Multiply2/1 -> Add1/3
  Cos/1 -> Multiply2/1
  beta/1 -> Sin/1, Cos1/1
  Sin2/1 -> Multiply1/2, Multiply/1
  Multiply/1 -> Add1/1
  MAS/1 -> Multiply1/1
  alpha/1 -> Sin2/1, Cos/1
  Cos1/1 -> Multiply/3
  LAS/1 -> Multiply/2
  Multiply1/1 -> Add1/2
  Add1/1 -> NAB/1

== system Poject_PilotInLoop_Beech_99_Nonlinear_Simulation_Altitude_hold/Airplane Dynamics/Euler's Angles (Phi,Theta,Psi)/PhiBlock ==
  P : Inport
  Q : Inport  Port=2
  Theta : Inport  Port=3
  R : Inport  Port=4
  Add : Sum  Inputs=+++
  Cos : Trigonometry  Operator=cos
  Integrator : Integrator
  Multiply : Product  Inputs=3
  Multiply1 : Product  Inputs=3
  Sin : Trigonometry
  Tan : Trigonometry  Operator=tan
  Phi : Outport
  wires:
  Multiply/1 -> Add/2
  Integrator/1 -> Sin/1, Cos/1, Phi/1
  Q/1 -> Multiply/1
  Tan/1 -> Multiply1/1, Multiply/3
  P/1 -> Add/1
  Add/1 -> Integrator/1
  Sin/1 -> Multiply/2
  Theta/1 -> Tan/1
  Cos/1 -> Multiply1/3
  R/1 -> Multiply1/2
  Multiply1/1 -> Add/3

== system Poject_PilotInLoop_Beech_99_Nonlinear_Simulation_Altitude_hold/Airplane Dynamics/Euler's Angles (Phi,Theta,Psi)/PsiBlock ==
  Q : Inport
  "Phi " : Inport  Port=2
  "Theta " : Inport  Port=3
  "R " : Inport  Port=4
  Add : Sum
  Cos : Trigonometry  Operator=cos
  Cos1 : Trigonometry  Operator=cos
  Divide1 : Product  Inputs=*/
  Divide2 : Product  Inputs=/*
  Integrator : Integrator
  Multiply : Product
  Multiply1 : Product
  Sin : Trigonometry
  Psi : Outport
  wires:
  "Phi "/1 -> Cos1/1, Sin/1
  Multiply1/1 -> Add/2
  Sin/1 -> Divide1/1
  Divide2/1 -> Multiply1/1
  Add/1 -> Integrator/1
  Q/1 -> Multiply/1
  Cos/1 -> Divide2/1, Divide1/2
  "R "/1 -> Multiply1/2
  Integrator/1 -> Psi/1
  Divide1/1 -> Multiply/2
  Cos1/1 -> Divide2/2
  "Theta "/1 -> Cos/1
  Multiply/1 -> Add/1

== system Poject_PilotInLoop_Beech_99_Nonlinear_Simulation_Altitude_hold/Airplane Dynamics/Euler's Angles (Phi,Theta,Psi)/ThetaBlock ==
  Phi : Inport
  R : Inport  Port=2
  Q : Inport  Port=3
  Add : Sum  Inputs=+-
  Cos : Trigonometry  Operator=cos
  Integrator : Integrator
  Multiply : Product
  Multiply1 : Product
  Sin : Trigonometry
  Theta : Outport
  wires:
  Multiply/1 -> Add/1
  Phi/1 -> Sin/1, Cos/1
  Q/1 -> Multiply/1
  Integrator/1 -> Theta/1
  Sin/1 -> Multiply1/1
  Multiply1/1 -> Add/2
  R/1 -> Multiply1/2
  Cos/1 -> Multiply/2
  Add/1 -> Integrator/1

== system Poject_PilotInLoop_Beech_99_Nonlinear_Simulation_Altitude_hold/Airplane Dynamics/Linear Velocities (U,V,W)/UBlock ==
  gx : Inport
  "FAxB " : Inport  Port=2
  "FTx " : Inport  Port=3
  "Q " : Inport  Port=4
  W : Inport  Port=5
  "R " : Inport  Port=6
  V : Inport  Port=7
  Add : Sum  Inputs=++-+
  Add1 : Sum
  "Aircraft Mass " : Constant  Value=mass  SampleTime=-1
  Divide1 : Product  Inputs=*/
  Integrator : Integrator  InitialCondition=450
  Multiply : Product
  Multiply1 : Product
  U : Outport
  wires:
  Integrator/1 -> U/1
  Multiply1/1 -> Add/4
  "Q "/1 -> Multiply/1
  Multiply/1 -> Add/3
  Divide1/1 -> Add/2
  "R "/1 -> Multiply1/1
  Add/1 -> Integrator/1
  W/1 -> Multiply/2
  V/1 -> Multiply1/2
  gx/1 -> Add/1
  Add1/1 -> Divide1/1
  "FAxB "/1 -> Add1/1
  "Aircraft Mass "/1 -> Divide1/2
  "FTx "/1 -> Add1/2

== system Poject_PilotInLoop_Beech_99_Nonlinear_Simulation_Altitude_hold/Airplane Dynamics/Linear Velocities (U,V,W)/VBlock ==
  gy : Inport
  "FAyB " : Inport  Port=2
  "FTy " : Inport  Port=3
  "U " : Inport  Port=4
  R : Inport  Port=5
  "P " : Inport  Port=6
  W : Inport  Port=7
  Add : Sum  Inputs=++-+
  Add1 : Sum
  Aircraft Mass : Constant  Value=mass  SampleTime=-1
  Divide1 : Product  Inputs=*/
  Integrator : Integrator
  Multiply : Product
  Multiply1 : Product
  V : Outport
  wires:
  "FTy "/1 -> Add1/2
  Aircraft Mass/1 -> Divide1/2
  "FAyB "/1 -> Add1/1
  Add1/1 -> Divide1/1
  gy/1 -> Add/1
  W/1 -> Multiply1/2
  R/1 -> Multiply/2
  Add/1 -> Integrator/1
  "P "/1 -> Multiply1/1
  Divide1/1 -> Add/2
  Multiply/1 -> Add/3
  "U "/1 -> Multiply/1
  Multiply1/1 -> Add/4
  Integrator/1 -> V/1

== system Poject_PilotInLoop_Beech_99_Nonlinear_Simulation_Altitude_hold/Airplane Dynamics/Linear Velocities (U,V,W)/WBlock ==
  gz : Inport
  "FAzB " : Inport  Port=2
  "FTz " : Inport  Port=3
  "P " : Inport  Port=4
  V : Inport  Port=5
  "Q " : Inport  Port=6
  "U " : Inport  Port=7
  Add : Sum  Inputs=++-+
  Add1 : Sum
  Aircraft Mass : Constant  Value=mass  SampleTime=-1
  Divide1 : Product  Inputs=*/
  Integrator : Integrator  InitialCondition=0.00031937779982
  Multiply : Product
  Multiply1 : Product
  W : Outport
  wires:
  Multiply1/1 -> Add/4
  "P "/1 -> Multiply/1
  Multiply/1 -> Add/3
  Divide1/1 -> Add/2
  "Q "/1 -> Multiply1/1
  Add/1 -> Integrator/1
  V/1 -> Multiply/2
  "U "/1 -> Multiply1/2
  gz/1 -> Add/1
  Add1/1 -> Divide1/1
  "FAzB "/1 -> Add1/1
  Aircraft Mass/1 -> Divide1/2
  "FTz "/1 -> Add1/2
  Integrator/1 -> W/1

== system Poject_PilotInLoop_Beech_99_Nonlinear_Simulation_Altitude_hold/Airplane Dynamics/Navigation/XInertiaBlock ==
  U : Inport
  V : Inport  Port=2
  W : Inport  Port=3
  Phi : Inport  Port=4
  Theta : Inport  Port=5
  Psi : Inport  Port=6
  Add1 : Sum  Inputs=+++
  Add2 : Sum  Inputs=-+
  Add3 : Sum
  Cos : Trigonometry  Operator=cos
  Cos1 : Trigonometry  Operator=cos
  Cos2 : Trigonometry  Operator=cos
  Integrator : Integrator
  Multiply : Product  Inputs=***
  Multiply1 : Product  Inputs=****
  Multiply2 : Product  Inputs=***
  Multiply3 : Product  Inputs=****
  Multiply4 : Product  Inputs=***
  Sin : Trigonometry
  Sin1 : Trigonometry
  Sin2 : Trigonometry
  To Workspace : ToWorkspace  VariableName=XdotInertia  SampleTime=-1
  XInertia : Outport
  wires:
  Integrator/1 -> XInertia/1
  Cos2/1 -> Multiply1/2, Multiply/2, Multiply3/2
  V/1 -> Multiply1/1, Multiply2/1
  Multiply1/1 -> Add2/2
  Sin2/1 -> Multiply2/3, Multiply4/2
  Psi/1 -> Cos2/1, Sin2/1
  Add3/1 -> Add1/3
  Multiply4/1 -> Add3/2
  Phi/1 -> Sin1/1, Cos/1
  Sin/1 -> Multiply1/3, Multiply3/3
  Cos/1 -> Multiply3/4, Multiply2/2
  Multiply/1 -> Add1/1
  Multiply3/1 -> Add3/1
  W/1 -> Multiply4/1, Multiply3/1
  Sin1/1 -> Multiply4/3, Multiply1/4
  Add1/1 -> To Workspace/1, Integrator/1
  Cos1/1 -> Multiply/3
  Theta/1 -> Sin/1, Cos1/1
  Multiply2/1 -> Add2/1
  U/1 -> Multiply/1
  Add2/1 -> Add1/2

== system Poject_PilotInLoop_Beech_99_Nonlinear_Simulation_Altitude_hold/Airplane Dynamics/Navigation/YInertiaBlock ==
  U : Inport
  V : Inport  Port=2
  W : Inport  Port=3
  Phi : Inport  Port=4
  Theta : Inport  Port=5
  Psi : Inport  Port=6
  Add1 : Sum  Inputs=+++
  Add2 : Sum
  Add3 : Sum  Inputs=+-
  Cos : Trigonometry  Operator=cos
  Cos1 : Trigonometry  Operator=cos
  Cos2 : Trigonometry  Operator=cos
  Integrator : Integrator
  Multiply : Product  Inputs=***
  Multiply1 : Product  Inputs=****
  Multiply2 : Product  Inputs=***
  Multiply3 : Product  Inputs=****
  Multiply4 : Product  Inputs=***
  Sin : Trigonometry
  Sin1 : Trigonometry
  Sin2 : Trigonometry
  To Workspace : ToWorkspace  VariableName=YdotInertia  SampleTime=-1
  YInertia : Outport
  wires:
  Add2/1 -> Add1/2
  U/1 -> Multiply/1
  Multiply2/1 -> Add2/1
  Theta/1 -> Sin/1, Cos1/1
  Cos1/1 -> Multiply/3
  Add1/1 -> To Workspace/1, Integrator/1
  Sin1/1 -> Multiply1/4, Multiply4/3
  W/1 -> Multiply3/1, Multiply4/1
  Multiply3/1 -> Add3/1
  Multiply/1 -> Add1/1
  Cos/1 -> Multiply3/4, Multiply2/2
  Sin/1 -> Multiply3/3, Multiply1/3
  Phi/1 -> Cos/1, Sin1/1
  Multiply4/1 -> Add3/2
  Add3/1 -> Add1/3
  Psi/1 -> Sin2/1, Cos2/1
  Sin2/1 -> Multiply3/2, Multiply/2, Multiply1/2
  Multiply1/1 -> Add2/2
  V/1 -> Multiply1/1, Multiply2/1
  Cos2/1 -> Multiply4/2, Multiply2/3
  Integrator/1 -> YInertia/1

== system Poject_PilotInLoop_Beech_99_Nonlinear_Simulation_Altitude_hold/Airplane Dynamics/Navigation/ZInertiaBlock ==
  U : Inport
  V : Inport  Port=2
  W : Inport  Port=3
  Phi : Inport  Port=4
  Theta : Inport  Port=5
  Add1 : Sum  Inputs=-++
  Cos : Trigonometry  Operator=cos
  Cos1 : Trigonometry  Operator=cos
  Integrator : Integrator  InitialCondition=-20000
  Multiply : Product
  Multiply1 : Product  Inputs=***
  Multiply2 : Product  Inputs=***
  Sin : Trigonometry
  Sin1 : Trigonometry
  To Workspace : ToWorkspace  VariableName=ZdotInertia  SampleTime=-1
  ZInertia : Outport
  wires:
  U/1 -> Multiply/1
  Theta/1 -> Cos/1, Sin/1
  Sin1/1 -> Multiply1/3
  Multiply2/1 -> Add1/3
  Cos/1 -> Multiply2/1, Multiply1/2
  Multiply1/1 -> Add1/2
  Phi/1 -> Cos1/1, Sin1/1
  Sin/1 -> Multiply/2
  Multiply/1 -> Add1/1
  W/1 -> Multiply2/3
  Cos1/1 -> Multiply2/2
  Add1/1 -> To Workspace/1, Integrator/1
  Integrator/1 -> ZInertia/1
  V/1 -> Multiply1/1

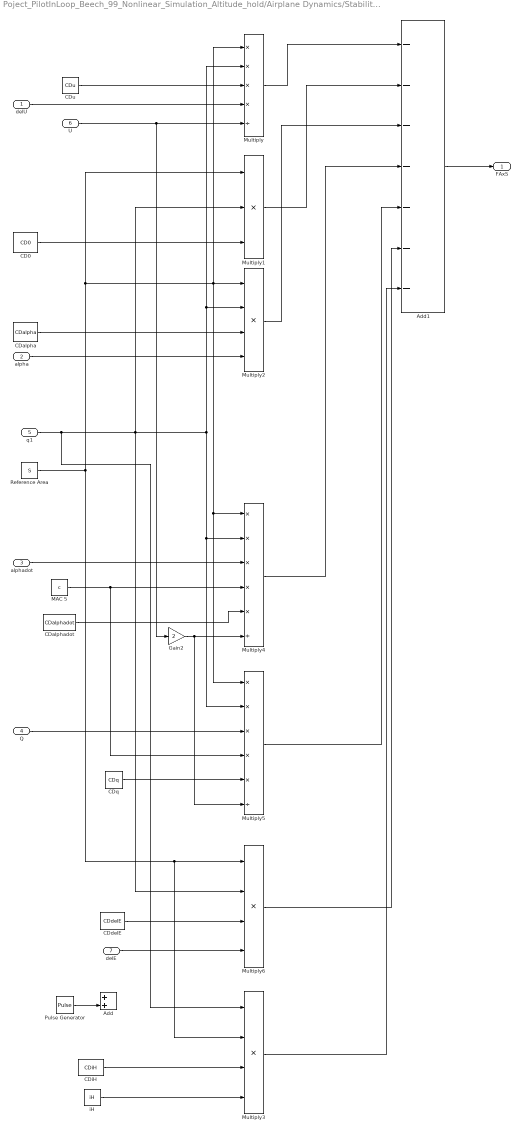
== system Poject_PilotInLoop_Beech_99_Nonlinear_Simulation_Altitude_hold/Airplane Dynamics/Stability Aerodunamic Forces and Moments (FAxS,FAyS,FAzS,LAS,MAS,NAS)/FAxSBlock ==
  delU : Inport
  alpha : Inport  Port=2
  alphadot : Inport  Port=3
  Q : Inport  Port=4
  q1 : Inport  Port=5
  U : Inport  Port=6
  delE : Inport  Port=7
  Add : Sum
  Add1 : Sum  Inputs=-------
  CD0 : Constant  Value=CD0
  CDalpha : Constant  Value=CDalpha
  CDalphadot : Constant  Value=CDalphadot
  CDdelE : Constant  Value=CDdelE
  CDiH : Constant  Value=CDiH
  CDq : Constant  Value=CDq
  CDu : Constant  Value=CDu
  Gain2 : Gain  Gain=2
  MAC 5 : Constant  Value=c
  Multiply : Product  Inputs=****/
  Multiply1 : Product  Inputs=***
  Multiply2 : Product  Inputs=****
  Multiply3 : Product  Inputs=****
  Multiply4 : Product  Inputs=*****/
  Multiply5 : Product  Inputs=*****/
  Multiply6 : Product  Inputs=****
  Pulse Generator : DiscretePulseGenerator  PulseType=Time based  Amplitude=0.035  Period=2000  PulseWidth=0.05
  "Reference Area " : Constant  Value=S
  iH : Constant  Value=iH
  FAxS : Outport
  wires:
  U/1 -> Gain2/1, Multiply/5
  q1/1 -> Multiply3/1, Multiply6/2, Multiply/2, Multiply2/2, Multiply5/2, Multiply4/2, Multiply1/2
  delU/1 -> Multiply/4
  "Reference Area "/1 -> Multiply/1, Multiply5/1, Multiply4/1, Multiply2/1, Multiply1/1, Multiply6/1, Multiply3/2
  alphadot/1 -> Multiply4/3
  Q/1 -> Multiply5/3
  MAC 5/1 -> Multiply4/4, Multiply5/4
  alpha/1 -> Multiply2/4
  Add1/1 -> FAxS/1
  Multiply/1 -> Add1/1
  CDq/1 -> Multiply5/5
  CDalphadot/1 -> Multiply4/5
  Multiply5/1 -> Add1/5
  Gain2/1 -> Multiply4/6, Multiply5/6
  Multiply2/1 -> Add1/3
  CDu/1 -> Multiply/3
  CDalpha/1 -> Multiply2/3
  CDdelE/1 -> Multiply6/3
  Multiply6/1 -> Add1/6
  Multiply4/1 -> Add1/4
  Multiply1/1 -> Add1/2
  CD0/1 -> Multiply1/3
  iH/1 -> Multiply3/4
  CDiH/1 -> Multiply3/3
  Multiply3/1 -> Add1/7
  delE/1 -> Multiply6/4
  Pulse Generator/1 -> Add/2

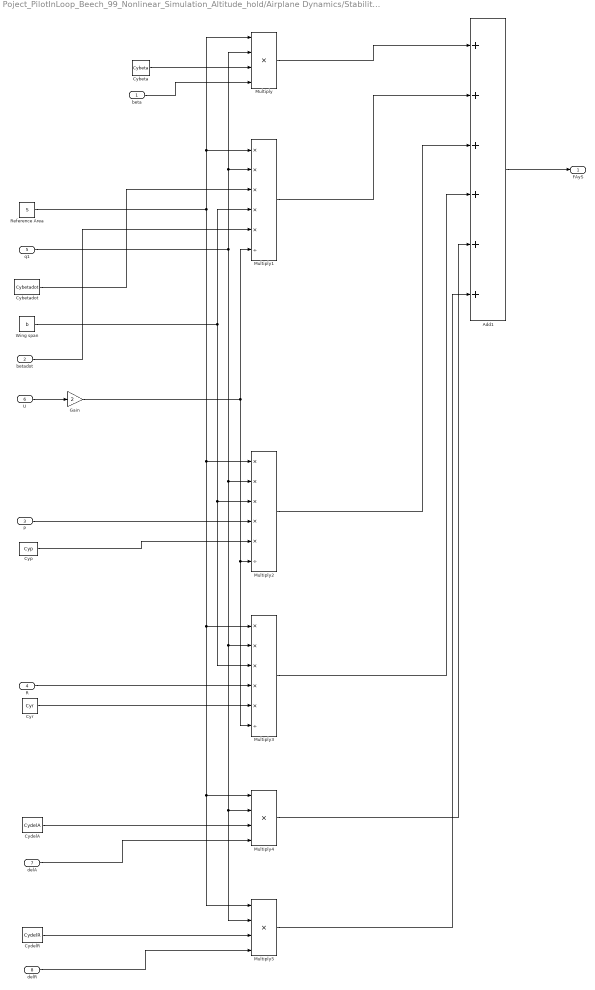
== system Poject_PilotInLoop_Beech_99_Nonlinear_Simulation_Altitude_hold/Airplane Dynamics/Stability Aerodunamic Forces and Moments (FAxS,FAyS,FAzS,LAS,MAS,NAS)/FAySBlock ==
  beta : Inport
  betadot : Inport  Port=2
  P : Inport  Port=3
  R : Inport  Port=4
  q1 : Inport  Port=5
  U : Inport  Port=6
  delA : Inport  Port=7
  delR : Inport  Port=8
  Add1 : Sum  Inputs=++++++
  Cybeta : Constant  Value=Cybeta
  Cybetadot : Constant  Value=Cybetadot
  CydelA : Constant  Value=CydelA
  CydelR : Constant  Value=CydelR
  Cyp : Constant  Value=Cyp
  Cyr : Constant  Value=Cyr
  Gain : Gain  Gain=2
  Multiply : Product  Inputs=****
  Multiply1 : Product  Inputs=*****/
  Multiply2 : Product  Inputs=*****/
  Multiply3 : Product  Inputs=*****/
  Multiply4 : Product  Inputs=****
  Multiply5 : Product  Inputs=****
  Reference Area : Constant  Value=S
  Wing span : Constant  Value=b
  FAyS : Outport
  wires:
  CydelR/1 -> Multiply5/3
  Cybetadot/1 -> Multiply1/3
  Multiply5/1 -> Add1/6
  Cyp/1 -> Multiply2/5
  Reference Area/1 -> Multiply5/1, Multiply4/1, Multiply3/1, Multiply2/1, Multiply/1, Multiply1/1
  Add1/1 -> FAyS/1
  Wing span/1 -> Multiply2/3, Multiply3/3, Multiply1/4
  betadot/1 -> Multiply1/5
  CydelA/1 -> Multiply4/3
  Gain/1 -> Multiply2/6, Multiply3/6, Multiply1/6
  q1/1 -> Multiply5/2, Multiply4/2, Multiply3/2, Multiply2/2, Multiply/2, Multiply1/2
  Multiply1/1 -> Add1/2
  delR/1 -> Multiply5/4
  P/1 -> Multiply2/4
  Multiply4/1 -> Add1/5
  R/1 -> Multiply3/4
  Cyr/1 -> Multiply3/5
  Multiply2/1 -> Add1/3
  beta/1 -> Multiply/4
  Multiply/1 -> Add1/1
  Cybeta/1 -> Multiply/3
  Multiply3/1 -> Add1/4
  U/1 -> Gain/1
  delA/1 -> Multiply4/4

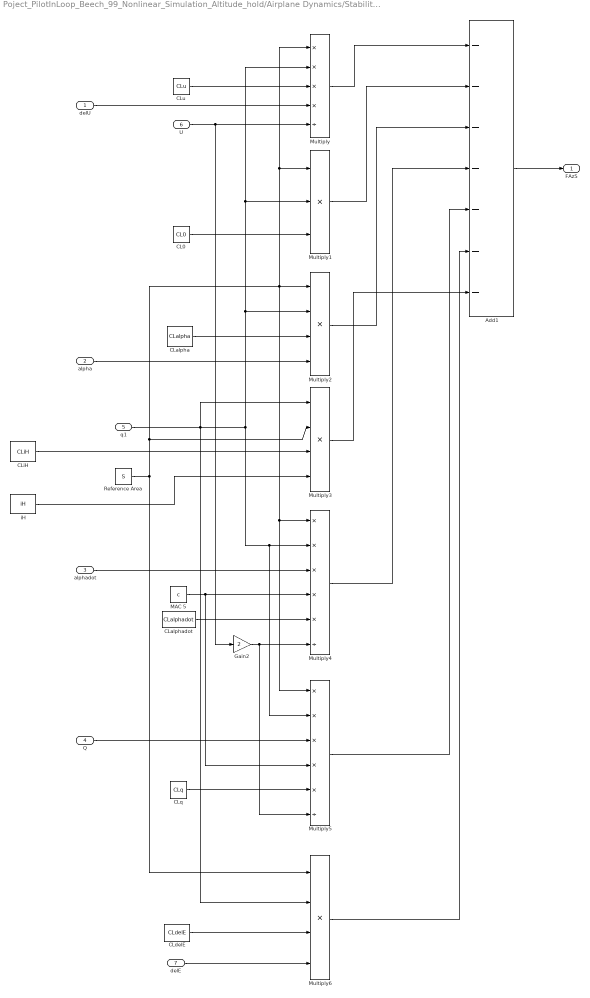
== system Poject_PilotInLoop_Beech_99_Nonlinear_Simulation_Altitude_hold/Airplane Dynamics/Stability Aerodunamic Forces and Moments (FAxS,FAyS,FAzS,LAS,MAS,NAS)/FAzSBlock ==
  delU : Inport
  alpha : Inport  Port=2
  alphadot : Inport  Port=3
  Q : Inport  Port=4
  q1 : Inport  Port=5
  U : Inport  Port=6
  delE : Inport  Port=7
  Add1 : Sum  Inputs=-------
  CL0 : Constant  Value=CL0
  CLalpha : Constant  Value=CLalpha
  CLalphadot : Constant  Value=CLalphadot
  CLdelE : Constant  Value=CLdelE
  CLiH : Constant  Value=CLiH
  CLq : Constant  Value=CLq
  CLu : Constant  Value=CLu
  Gain2 : Gain  Gain=2
  MAC 5 : Constant  Value=c
  Multiply : Product  Inputs=****/
  Multiply1 : Product  Inputs=***
  Multiply2 : Product  Inputs=****
  Multiply3 : Product  Inputs=****
  Multiply4 : Product  Inputs=*****/
  Multiply5 : Product  Inputs=*****/
  Multiply6 : Product  Inputs=****
  "Reference Area " : Constant  Value=S
  iH : Constant  Value=iH
  FAzS : Outport
  wires:
  CL0/1 -> Multiply1/3
  Multiply4/1 -> Add1/4
  Multiply6/1 -> Add1/6
  CLdelE/1 -> Multiply6/3
  CLalpha/1 -> Multiply2/3
  CLu/1 -> Multiply/3
  Multiply2/1 -> Add1/3
  Multiply1/1 -> Add1/2
  Gain2/1 -> Multiply5/6, Multiply4/6
  Multiply5/1 -> Add1/5
  CLalphadot/1 -> Multiply4/5
  CLq/1 -> Multiply5/5
  Multiply/1 -> Add1/1
  Add1/1 -> FAzS/1
  alpha/1 -> Multiply2/4
  MAC 5/1 -> Multiply5/4, Multiply4/4
  Q/1 -> Multiply5/3
  alphadot/1 -> Multiply4/3
  "Reference Area "/1 -> Multiply2/1, Multiply4/1, Multiply5/1, Multiply/1, Multiply1/1, Multiply3/2, Multiply6/1
  delU/1 -> Multiply/4
  q1/1 -> Multiply6/2, Multiply4/2, Multiply5/2, Multiply2/2, Multiply1/2, Multiply/2, Multiply3/1
  U/1 -> Multiply/5, Gain2/1
  CLiH/1 -> Multiply3/3
  iH/1 -> Multiply3/4
  Multiply3/1 -> Add1/7
  delE/1 -> Multiply6/4
